simulink model "testrl"  (R2019b)
settings: Solver=VariableStepAuto  StartTime=0.0  StopTime=20  RelTol=1e-3
undefined symbols (not defined in the file or in its folder): rl
libraries: rllib x1, simulink x1, powerlib x1
settings Model: Creator=conqu  LastModifiedBy=conqu

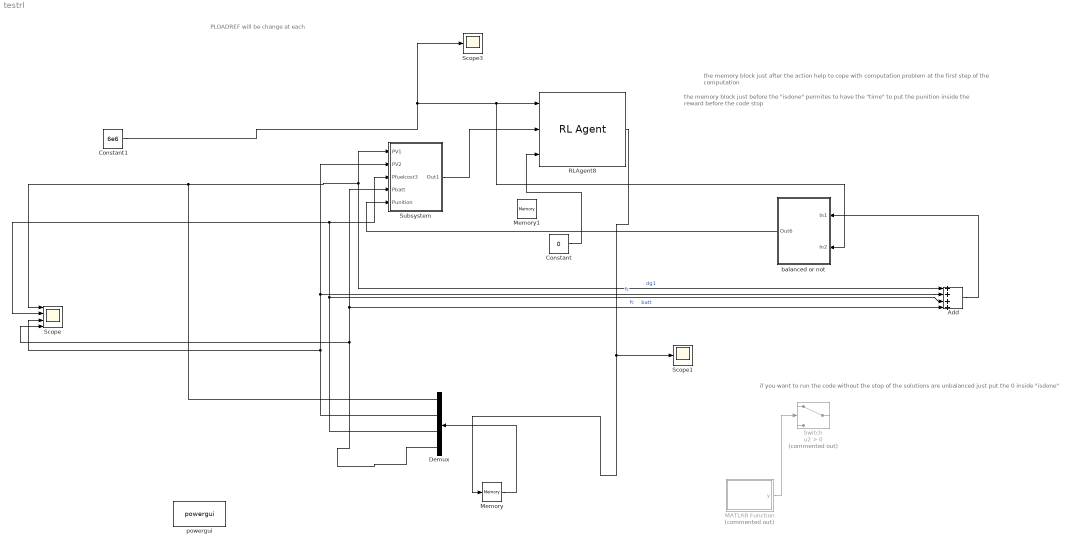
== system testrl ==
  note: PLOADREF will be change at each
  note: if you want to run the code without the stop of the solutions are unbalanced just put the 0 inside "isdone"
  note: the memory block just after the action help to cope with computation problem at the first step of the computation
  note: the memory block just before the "isdone" permites to have the "time" to put the punition inside the reward before the code stop
  Add : Sum  Inputs=++++
  Constant : Constant  Value=0
  Constant1 : Constant  Value=6e6
  Demux : Demux
  MATLAB Function : MATLAB Function  Commented=on  TreatAsAtomicUnit=on
  Memory : Memory  InheritSampleTime=on  LinearizeAsDelay=on
  Memory1 : Memory
  RLAgent8 : rllib/RL Agent  Agent=rl.util.PolicyInstance.get()  ProvideReward=on  ProvideIsDone=on  ProvideCumRwd=off  TreatAsDirectFeedthrough=on  CollectLoggedSignals=on  CollectModelStates=on
      settings: SourceProductName=Reinforcement Learning Toolbox
  Scope : Scope  NumInputPorts=4
  Scope1 : Scope
  Scope3 : Scope
  Subsystem : Subsystem
  Switch : Switch  Commented=on  Criteria=u2 > Threshold
  "balanced or not " : Subsystem
  powergui : powerlib/powergui  Priority=1  SimulationMode=Discrete  SampleTime=0.1  frequency=60  Iterations=50  frequencyindice=60  Pbase=100e6  ErrMax=1e-4  UnitsV=kV  UnitsW=MW  buscounter=0  FunctionMessages=off  echomessages=off  EnableUseOfTLC=off  CurrentSourceSwitches=off  DisableSnubberDevices=off  DisableRonSwitches=off  DisableVfSwitches=off  DisplayEquations=off  AutomaticDiscreteSolvers=off  SolverType=Tustin/Backward Euler (TBE)  Interpol=off  ExternalGateDelay=off  methode=off  Ts=100  x0status=blocks  SPID=on  SwTol=0  HookPort=off  NonlinearTolerance=1e-4  nMaxIteration=100  ContinueOnMaxIteration=off  RestoreLinks=warning  ResistiveCurrentMeasurement=off  Frange=[0:2:500]  Ylog=off  Xlog=on  ShowGrid=off  save=off  variable=ZData  structure=0  ZoomFFT=off  StartTime=0.0  cycles=1  DisplayStyle=1  fundamental=60  FreqAxis=off  MaxFrequency=1000  frequencyindicesteady=1  RmsSteady=1  display=off
      settings: SourceProductName=Simscape Electrical
  wires:
  Demux/2 -> Add/2, Subsystem/2(PV2), Scope/3  "fc"
  Subsystem/1(Out1) -> RLAgent8/2
  Demux/1 -> Add/1, Subsystem/1(PV1), Scope/1  "dg1"
  RLAgent8/1 -> Memory/1, Scope1/1
  Demux/3 -> Scope/2, Subsystem/3(Pfuelcost3), Add/3  "fc"
  Constant/1 -> RLAgent8/3
  Demux/4 -> Subsystem/4("Pbatt "), Add/4, Scope/4  "batt"
  Constant1/1 -> Scope3/1, "balanced or not "/2(In2), RLAgent8/1
  "balanced or not "/1(Out6) -> Subsystem/5(Punition)
  Add/1 -> "balanced or not "/1(In1)
  MATLAB Function/1(y) -> Switch/2
  Memory/1 -> Demux/1

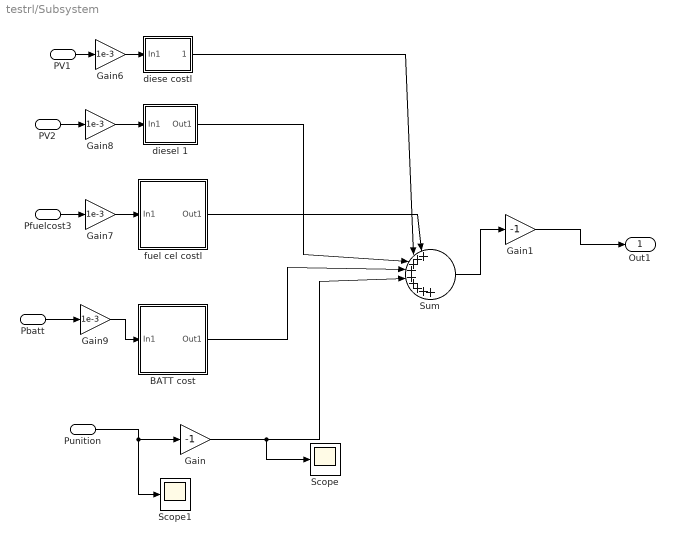
== system testrl/Subsystem ==
  PV1 : Inport
  PV2 : Inport  Port=2
  Pfuelcost3 : Inport  Port=3
  "Pbatt " : Inport  Port=4
  Punition : Inport  Port=5
  "BATT cost " : Subsystem
  Gain : Gain  Gain=-1
  Gain1 : Gain  Gain=-1
  Gain{6..9} (4 alike) : Gain  Gain=1e-3
  Scope : Scope
  Scope1 : Scope
  Sum : Sum  Inputs=|+++++++++
  "diese costl " : Subsystem
  diesel 1 : Subsystem
  "fuel cel costl " : Subsystem
  Out1 : Outport
  wires:
  PV1/1 -> Gain6/1
  "fuel cel costl "/1(Out1) -> Sum/1
  "diese costl "/1(Out1) -> Sum/2
  diesel 1/1(Out1) -> Sum/3
  "BATT cost "/1(Out1) -> Sum/4
  PV2/1 -> Gain8/1
  Pfuelcost3/1 -> Gain7/1
  Sum/1 -> Gain1/1
  Gain1/1 -> Out1/1
  "Pbatt "/1 -> Gain9/1
  Gain6/1 -> "diese costl "/1(In1)
  Gain8/1 -> diesel 1/1(In1)
  Gain7/1 -> "fuel cel costl "/1(In1)
  Gain9/1 -> "BATT cost "/1(In1)
  Punition/1 -> Scope1/1, Gain/1
  Gain/1 -> Scope/1, Sum/5

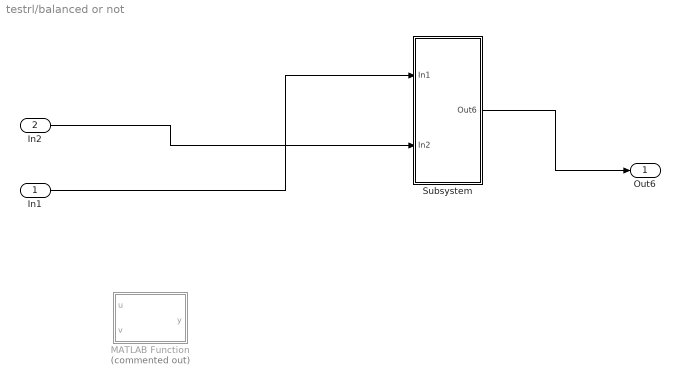
== system testrl/balanced or not  ==
  In1 : Inport
  In2 : Inport  Port=2
  MATLAB Function : MATLAB Function  Commented=on  TreatAsAtomicUnit=on
  Subsystem : Subsystem
  Out6 : Outport
  wires:
  In2/1 -> Subsystem/2(In2)
  In1/1 -> Subsystem/1(In1)
  Subsystem/1(Out6) -> Out6/1

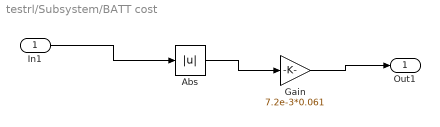
== system testrl/Subsystem/BATT cost  ==
  In1 : Inport
  Abs : Abs
  Gain : Gain  Gain=7.2e-3*0.061
  Out1 : Outport
  wires:
  In1/1 -> Abs/1
  Abs/1 -> Gain/1
  Gain/1 -> Out1/1

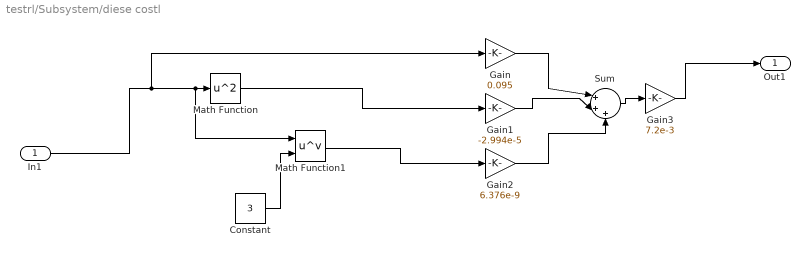
== system testrl/Subsystem/diese costl  ==
  In1 : Inport
  Constant : Constant  Value=3
  Gain : Gain  Gain=0.095
  Gain1 : Gain  Gain=-2.994e-5
  Gain2 : Gain  Gain=6.376e-9
  Gain3 : Gain  Gain=7.2e-3
  Math Function : Math  Operator=square  SignedPower=off  SaturateOnIntegerOverflow=on
  Math Function1 : Math  Operator=pow  SignedPower=off  SaturateOnIntegerOverflow=on
  Sum : Sum  Inputs=|+++
  Out1 : Outport
  wires:
  Sum/1 -> Gain3/1
  Constant/1 -> Math Function1/2
  Math Function1/1 -> Gain2/1
  Math Function/1 -> Gain1/1
  In1/1 -> Gain/1, Math Function1/1, Math Function/1
  Gain/1 -> Sum/1
  Gain2/1 -> Sum/3
  Gain1/1 -> Sum/2
  Gain3/1 -> Out1/1

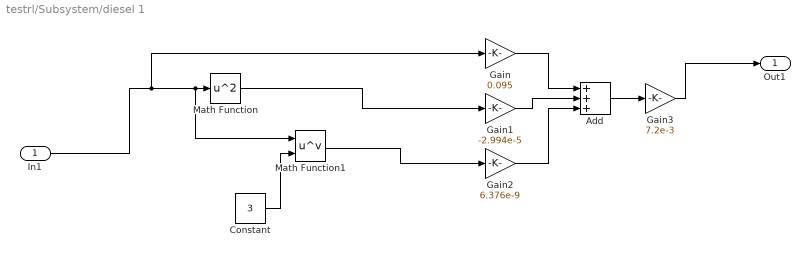
== system testrl/Subsystem/diesel 1 ==
  In1 : Inport
  Add : Sum  Inputs=+++
  Constant : Constant  Value=3
  Gain : Gain  Gain=0.095
  Gain1 : Gain  Gain=-2.994e-5
  Gain2 : Gain  Gain=6.376e-9
  Gain3 : Gain  Gain=7.2e-3
  Math Function : Math  Operator=square  SignedPower=off  SaturateOnIntegerOverflow=on
  Math Function1 : Math  Operator=pow  SignedPower=off  SaturateOnIntegerOverflow=on
  Out1 : Outport
  wires:
  Add/1 -> Gain3/1
  Constant/1 -> Math Function1/2
  Math Function1/1 -> Gain2/1
  Math Function/1 -> Gain1/1
  In1/1 -> Gain/1, Math Function1/1, Math Function/1
  Gain/1 -> Add/1
  Gain2/1 -> Add/3
  Gain1/1 -> Add/2
  Gain3/1 -> Out1/1

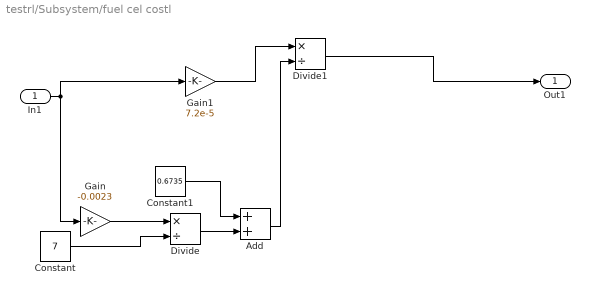
== system testrl/Subsystem/fuel cel costl  ==
  In1 : Inport
  Add : Sum
  Constant : Constant  Value=7
  Constant1 : Constant  Value=0.6735
  Divide : Product  Inputs=*/
  Divide1 : Product  Inputs=*/
  Gain : Gain  Gain=-0.0023
  Gain1 : Gain  Gain=7.2e-5
  Out1 : Outport
  wires:
  In1/1 -> Gain1/1, Gain/1
  Constant/1 -> Divide/2
  Gain/1 -> Divide/1
  Divide/1 -> Add/2
  Constant1/1 -> Add/1
  Add/1 -> Divide1/2
  Gain1/1 -> Divide1/1
  Divide1/1 -> Out1/1

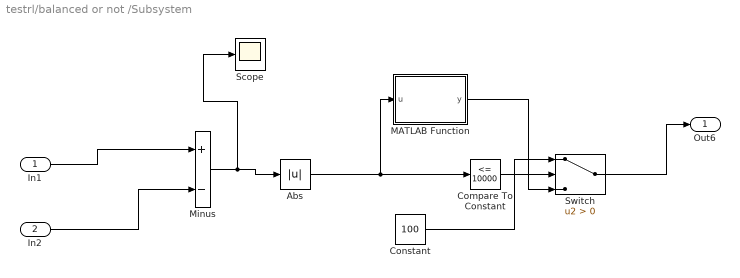
== system testrl/balanced or not /Subsystem ==
  In1 : Inport
  In2 : Inport  Port=2
  Abs : Abs
  Compare To Constant : simulink/Logic and Bit Operations/Compare To Constant  relop=<=  const=10000  OutDataTypeStr=boolean
  Constant : Constant  Value=100
  MATLAB Function : MATLAB Function  TreatAsAtomicUnit=on
  Minus : Sum  Inputs=+-
  Scope : Scope
  Switch : Switch  Criteria=u2 > Threshold
  Out6 : Outport
  wires:
  In1/1 -> Minus/1
  Abs/1 -> MATLAB Function/1(u), Compare To Constant/1
  In2/1 -> Minus/2
  Minus/1 -> Scope/1, Abs/1
  Switch/1 -> Out6/1
  Compare To Constant/1 -> Switch/2
  MATLAB Function/1(y) -> Switch/3
  Constant/1 -> Switch/1

== matlab function testrl/balanced or not /Subsystem/MATLAB Function ==
  data: u input; y output
function y = fcn(u)
valeur=-0.000555*u+105.555
y = valeur;

== matlab function testrl/balanced or not /MATLAB Function ==
  data: u input size=[4,1]; y output size=1; v input size=1
function y = fcn(u,v)
a=abs(u(1)+u(2)+u(4)+u(3)-v)
if a<=1000
    valeur=100
else
    valeur=-0.001*a+110
y = valeur;

== matlab function testrl/MATLAB Function ==
  data: y output
function y = fcn()
persistent i
if isempty(i)
    i=-1
end
i=i+1
u=i
y = u;
